simulink model "CubeSatOrbitSensitivitysim"  (R2026a)
settings: Solver=ode45  StopTime=tFinal  MaxStep=10.0  RelTol=1e-10  AbsTol=1e-6
values from neighbouring files (symbols this model uses):
  x0 = [r0; v0]    [Run_sweep.m]    (also in init_orbital.m)
settings Model: Creator=Sriram Dorai  LastModifiedBy=Sriram Dorai

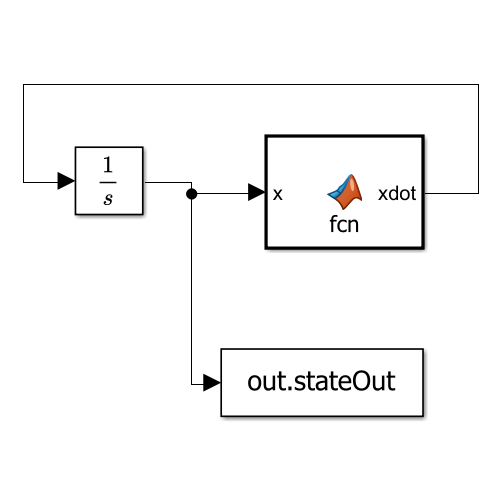
[thumbnail: Simulink's stored preview of the top-level diagram]
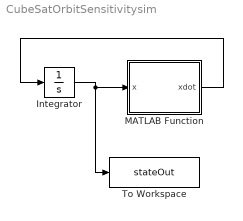
== system CubeSatOrbitSensitivitysim ==
  Integrator : Integrator  InitialCondition=x0
  MATLAB Function : MATLAB Function  TreatAsAtomicUnit=on
  To Workspace : ToWorkspace  VariableName=stateOut  SaveFormat=Timeseries  SampleTime=-1
  wires:
  Integrator/1 -> To Workspace/1, MATLAB Function/1(x)
  MATLAB Function/1(xdot) -> Integrator/1

== matlab function CubeSatOrbitSensitivitysim/MATLAB Function ==
  data: xdot output size=[6 1]; x input size=[6 1]
function xdot  = fcn(x)

mu = 3.986004418e14;  % m^3/s^2

r = x(1:3);           % position, m
v = x(4:6);           % velocity, m/s

rMag = sqrt(sum(r.^2));

% Two-body gravitational acceleration
a = -mu * r / rMag^3;

% State derivative: [position derivative; velocity derivative]
xdot = [v; a];

end
